simulink model "rotation"  (R2019a)
settings: Solver=VariableStepAuto  StartTime=0.0  StopTime=999  FixedStep=0.01  RelTol=1e-3
libraries: vrlib x1
settings Model: Creator=user  LastModifiedBy=Cal__
settings DataIOCC: ReturnWorkspaceOutputs=off
settings DebuggingCC: ArithmeticOperatorsInVariantConditions=warning

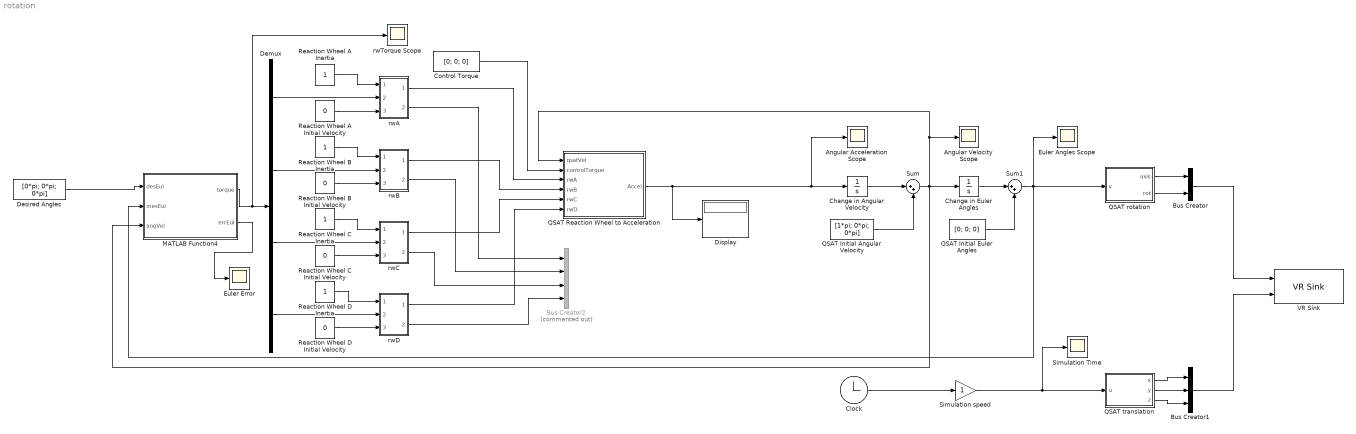
== system rotation ==
  Angular Acceleration Scope : Scope
  Angular Velocity Scope : Scope
  Bus Creator : BusCreator  Inputs=2
  Bus Creator1 : BusCreator  Inputs=3
  Bus Creator2 : BusCreator  Commented=on  Inputs=4
  Change in Angular Velocity : Integrator
  Change in Euler Angles : Integrator
  "Clock " : Clock
  Control Torque : Constant  Value=[0; 0; 0]
  Demux : Demux
  Desired Angles : Constant  Value=[0*pi; 0*pi; 0*pi]
  Display : Display
  Euler Angles Scope : Scope
  Euler Error : Scope
  MATLAB Function4 : MATLAB Function  TreatAsAtomicUnit=on
  QSAT Initial Angular Velocity : Constant  Value=[1*pi; 0*pi; 0*pi]
  QSAT Initial Euler Angles : Constant  Value=[0; 0; 0]
  QSAT Reaction Wheel to Acceleration : MATLAB Function  TreatAsAtomicUnit=on
  QSAT rotation : MATLAB Function  TreatAsAtomicUnit=on
  "QSAT translation " : MATLAB Function  TreatAsAtomicUnit=on
  Reaction Wheel A Inertia : Constant
  Reaction Wheel A Initial Velocity : Constant  Value=0
  Reaction Wheel B Inertia : Constant
  Reaction Wheel B Initial Velocity : Constant  Value=0
  Reaction Wheel C Inertia : Constant
  Reaction Wheel C Initial Velocity : Constant  Value=0
  Reaction Wheel D Inertia : Constant
  Reaction Wheel D Initial Velocity : Constant  Value=0
  "Simulation Time " : Scope
  Simulation speed : Gain
  Sum : Sum  Inputs=|++
  Sum1 : Sum  Inputs=|++
  VR Sink : vrlib/VR Sink  InstantiateOnLoad=on  SampleTime=0.1  ViewEnable=on  RemoteChange=off  RemoteView=off  FieldsWritten=STLB_transform.rotation.4.1.1.double#STLB_transform.translation.3.1.1.double  WorldFileName=world.wrl  AutoView=on  VideoDimensions=[]  AllowVariableSize=off  FigureProperties="{'Position', 'Name', 'Viewpoint', 'CameraBound', 'CameraDirection', 'CameraPosition', 'CameraUpVector', 'ZoomFactor', 'Antialiasing', 'Headlight', 'Lighting', 'NavPanel', 'Sound', 'StatusBar', 'Stereo3D', 'Stereo3DCameraOffset', 'Stereo3DHIT', 'ToolBar', 'Textures', 'Transparency', 'Triad', 'Wireframe', 'NavZones', 'NavMode', 'NavSpeed', 'CaptureFileFormat', 'CaptureFileName', 'Record2DCompressMethod', 'Record2DCompressQuality', 'Record2D', 'Record2DFileName', 'Record2DFPS'; [6.4166666666666663e+02   7.9000000000000114e+01   6.3866666666666663e+02   5.4933333333333326e+02], '', '_untitled_1', 'on', [0.0000000000000000e+00   0.0000000000000000e+00  -1.0000000000000000e+00], [0.0000000000000000e+00   0.0000000000000000e+00   0.0000000000000000e+00], [0.0000000000000000e+00   1.0000000000000000e+00   0.0000000000000000e+00], [1.0000000000000000e+00], 'on', 'on', 'on', 'halfbar', 'on', 'on', 'off', [1.0000000149011612e-01], [0.0000000000000000e+00], 'on', 'on', 'on', 'none', 'off', 'off', 'fly', 'normal', 'tif', '%f_anim_%n.tif', 'auto', [7.5000000000000000e+01], 'off', '%f_anim_%n.avi', 'auto'}"
      settings: SourceProductBaseCode=VR
  rwA : Subsystem
  rwB : Subsystem
  rwC : Subsystem
  rwD : Subsystem
  rwTorque Scope : Scope
  wires:
  MATLAB Function4/1(torque) -> rwTorque Scope/1, Demux/1
  QSAT Reaction Wheel to Acceleration/1(Accel) -> Display/1, Angular Acceleration Scope/1, Change in Angular Velocity/1
  "QSAT translation "/1(x) -> Bus Creator1/1
  QSAT Initial Euler Angles/1 -> Sum1/2
  Change in Euler Angles/1 -> Sum1/1
  Change in Angular Velocity/1 -> Sum/1
  QSAT Initial Angular Velocity/1 -> Sum/2
  Control Torque/1 -> QSAT Reaction Wheel to Acceleration/2(controlTorque)
  QSAT rotation/2(rot) -> Bus Creator/2
  Simulation speed/1 -> "Simulation Time "/1, "QSAT translation "/1(u)
  "QSAT translation "/3(z) -> Bus Creator1/3
  "QSAT translation "/2(y) -> Bus Creator1/2
  "Clock "/1 -> Simulation speed/1
  QSAT rotation/1(axis) -> Bus Creator/1
  rwA/1(rwA) -> QSAT Reaction Wheel to Acceleration/3(rwA)
  Reaction Wheel A Inertia/1 -> rwA/1(In1)
  Demux/1 -> rwA/2(In2)
  Reaction Wheel A Initial Velocity/1 -> rwA/3(In3)
  rwB/1(rwB) -> QSAT Reaction Wheel to Acceleration/4(rwB)
  Reaction Wheel B Inertia/1 -> rwB/1(In1)
  Demux/2 -> rwB/2(In2)
  Reaction Wheel B Initial Velocity/1 -> rwB/3(In3)
  rwC/1(rwC) -> QSAT Reaction Wheel to Acceleration/5(rwC)
  Demux/3 -> rwC/2(In2)
  Reaction Wheel C Initial Velocity/1 -> rwC/3(In3)
  rwD/1(rwD) -> QSAT Reaction Wheel to Acceleration/6(rwD)
  Demux/4 -> rwD/2(In2)
  Reaction Wheel D Initial Velocity/1 -> rwD/3(In3)
  Reaction Wheel C Inertia/1 -> rwC/1(In1)
  Reaction Wheel D Inertia/1 -> rwD/1(In1)
  rwA/2(VelA) -> Bus Creator2/1
  rwB/2(VelB) -> Bus Creator2/2
  rwC/2(VelC) -> Bus Creator2/3
  rwD/2(VelD) -> Bus Creator2/4
  Desired Angles/1 -> MATLAB Function4/1(desEul)
  Sum1/1 -> MATLAB Function4/2(mesEul), Euler Angles Scope/1, QSAT rotation/1(v)
  MATLAB Function4/2(errEul) -> Euler Error/1
  Sum/1 -> MATLAB Function4/3(angVel), Angular Velocity Scope/1, QSAT Reaction Wheel to Acceleration/1(qsatVel), Change in Euler Angles/1
  Bus Creator/1 -> VR Sink/1
  Bus Creator1/1 -> VR Sink/2

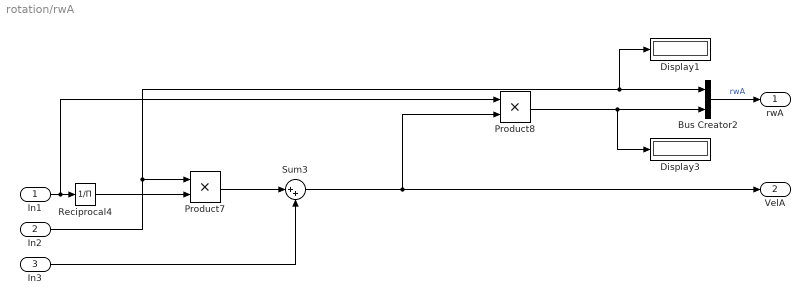
== system rotation/rwA ==
  In1 : Inport
  In2 : Inport  Port=2
  In3 : Inport  Port=3
  Bus Creator2 : BusCreator  Inputs=2
  Display1 : Display
  Display3 : Display
  Product7 : Product
  Product8 : Product
  Reciprocal4 : Product  Inputs=/
  Sum3 : Sum  Inputs=|++
  rwA : Outport
  VelA : Outport  Port=2
  wires:
  In2/1 -> Display1/1, Bus Creator2/1, Product7/1
  Product7/1 -> Sum3/1
  Product8/1 -> Display3/1, Bus Creator2/2
  Sum3/1 -> VelA/1, Product8/2
  In1/1 -> Product8/1, Reciprocal4/1
  Bus Creator2/1 -> rwA/1  "rwA"
  Reciprocal4/1 -> Product7/2
  In3/1 -> Sum3/2

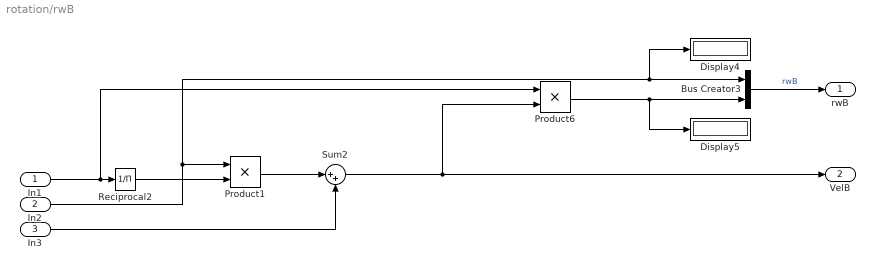
== system rotation/rwB ==
  In1 : Inport
  In2 : Inport  Port=2
  In3 : Inport  Port=3
  Bus Creator3 : BusCreator  Inputs=2
  Display4 : Display
  Display5 : Display
  Product1 : Product
  Product6 : Product
  Reciprocal2 : Product  Inputs=/
  Sum2 : Sum  Inputs=|++
  rwB : Outport
  VelB : Outport  Port=2
  wires:
  Reciprocal2/1 -> Product1/2
  In2/1 -> Display4/1, Bus Creator3/1, Product1/1
  In3/1 -> Sum2/2
  In1/1 -> Product6/1, Reciprocal2/1
  Product6/1 -> Display5/1, Bus Creator3/2
  Product1/1 -> Sum2/1
  Bus Creator3/1 -> rwB/1  "rwB"
  Sum2/1 -> VelB/1, Product6/2

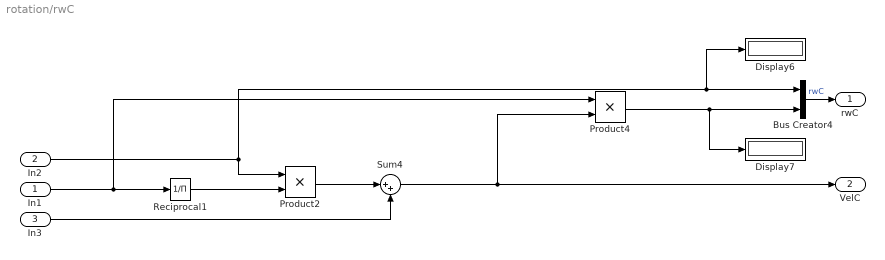
== system rotation/rwC ==
  In1 : Inport
  In2 : Inport  Port=2
  In3 : Inport  Port=3
  Bus Creator4 : BusCreator  Inputs=2
  Display6 : Display
  Display7 : Display
  Product2 : Product
  Product4 : Product
  Reciprocal1 : Product  Inputs=/
  Sum4 : Sum  Inputs=|++
  rwC : Outport
  VelC : Outport  Port=2
  wires:
  Product4/1 -> Display7/1, Bus Creator4/2
  Product2/1 -> Sum4/1
  Reciprocal1/1 -> Product2/2
  In3/1 -> Sum4/2
  Bus Creator4/1 -> rwC/1  "rwC"
  In2/1 -> Display6/1, Bus Creator4/1, Product2/1
  In1/1 -> Product4/1, Reciprocal1/1
  Sum4/1 -> Product4/2, VelC/1

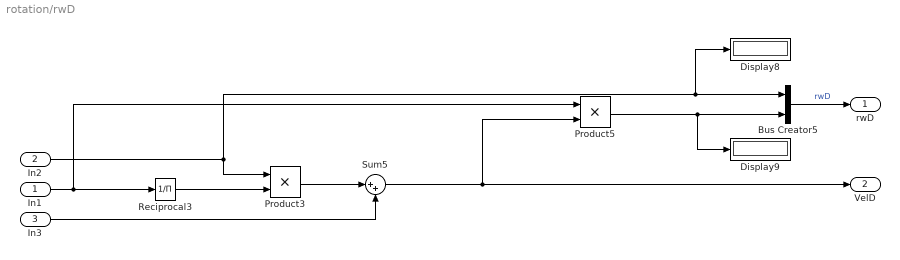
== system rotation/rwD ==
  In1 : Inport
  In2 : Inport  Port=2
  In3 : Inport  Port=3
  Bus Creator5 : BusCreator  Inputs=2
  Display8 : Display
  Display9 : Display
  Product3 : Product
  Product5 : Product
  Reciprocal3 : Product  Inputs=/
  Sum5 : Sum  Inputs=|++
  rwD : Outport
  VelD : Outport  Port=2
  wires:
  Product3/1 -> Sum5/1
  Reciprocal3/1 -> Product3/2
  Product5/1 -> Display9/1, Bus Creator5/2
  In3/1 -> Sum5/2
  Bus Creator5/1 -> rwD/1  "rwD"
  In2/1 -> Display8/1, Bus Creator5/1, Product3/1
  In1/1 -> Product5/1, Reciprocal3/1
  Sum5/1 -> VelD/1, Product5/2

== matlab function rotation/QSAT translation  ==
  data: x output; u input; y output; z output
function [x,y,z] = fcn(u)
    x=0;
    y=0;
    z=0;
end

== matlab function rotation/QSAT rotation ==
  data: axis output; v input; rot output
function [axis,rot] = fcn(v)
    
    %setup for manipulation
    cx = cos(v(1)/2);
    cy = cos(v(2)/2);
    cz = cos(v(3)/2);
    
    sx = sin(v(1)/2);
    sy = sin(v(2)/2);
    sz = sin(v(3)/2);
    
    %axis calculation
    x = sx*sy*cz + cx*cy*sz;
    y = sx*cy*cz + cx*sy*sz;
    z = cx*sy*cz - sx*cy*sz;
    
    axis = [x, y, z];
    
    %magnitude calculation
    rot = 2*acos(cx*cy*cz - sx*sy*sz);
end

== matlab function rotation/QSAT Reaction Wheel to Acceleration ==
  data: qsatVel input; controlTorque input; Accel output; rwA input; rwB input; rwC input; rwD input
function Accel = fcn(qsatVel, controlTorque, rwA, rwB, rwC, rwD)
%where each rw is a vector containing momentum and torque along the wheel's axis (elevation assumed to be pi/4)
    %rwA is on x
    %rwB is on y
    %rwC is on -x
    %rwD is on -y
    
%find ReactionWheel momentum and torque with respect to cubeSat coordinates
    a = cos(pi/4); %as cos(pi/4) == sin(pi/4)
    x = [0,0];
    y = [0,0];
    z = [0,0];
    for i = 1 : 2
        x(i) = a*(rwA(i) - rwC(i));
        y(i) = a*(rwB(i) - rwD(i));
        z(i) = a*(rwA(i) + rwB(i) + rwC(i) + rwD(i));
    end
    rwMomentum = [x(1); y(1); z(1)];
    rwTorque = [x(2); y(2); z(2)];
    
%find acceleration due to controller, reaction wheel, and cubeSat properties
    qsatInertia = [2.5000,      0,       0;
                        0, 2.5000,       0;
                        0,      0, 12.5000];
    qsatVelocity = qsatVel;
    %manipulation for equation
    invI = inv(qsatInertia);
    crossVel = [             0, -qsatVelocity(3), qsatVelocity(2);
               qsatVelocity(3),                0,-qsatVelocity(1);
              -qsatVelocity(2),  qsatVelocity(1),              0];            
    Hw = rwMomentum;
    Tw = rwTorque;
    Tc = controlTorque;
    %acceleration equation      
    Accel = -invI*crossVel*qsatInertia*qsatVelocity-invI*crossVel*Hw-invI*Tw-invI*Tc;

    %vel*t + accel*t*t

== matlab function rotation/MATLAB Function4 ==
  data: desEul input; torque output; mesEul input; errEul output; angVel input
function [torque, errEul] = RotationConversion(desEul, mesEul, angVel)

    angVelEul = angVel*20;
    %placeholder for integral
    
    mesEul = mod(mesEul, [2*pi;2*pi;2*pi]);
    for i = 1 : 3
        if mesEul(i) > 1.25*pi
            mesEul(i) = mesEul(i) - 2*pi;
        elseif mesEul(i) < -1.25*pi
            mesEul(i) = mesEul(i) + 2*pi;
        end
    end
    %removes extra rotations based on previous turns
    
    errEul = -.1*(desEul - mesEul - angVelEul);
    
    errWA = errEul(1);
    errWB = (errEul(3) - errEul(1) + errEul(2))/2;
    errWC = 0;
    errWD = errWB - errEul(2);
    %only 3 reaction wheels are needed
    
    temp = [errWA, errWB, errWC, errWD];
    torque = temp;
    
end
